simulink library "lib_methods"  (Simulink 7.7)
settings: Solver=ode45  StartTime=0.0  StopTime=10.0  RelTol=1e-3
undefined symbols (not defined in the file): AOBC_dt, DiscIntNeverNeededParam, dt, I, mom_lim, MTQ_out, Ratelim, RW_J, target_mom, three_one_skew_matrix, UT1_UTC
libraries: aerolibutil x15, lib_util x15, vrlib x4, lib_astrodynamics x3, aerolibtransform2 x1, lib_methods x1, lib_env x1
(part 1 of 2)
settings Model: Creator=miyata  LastModifiedBy=yamaurashusaku

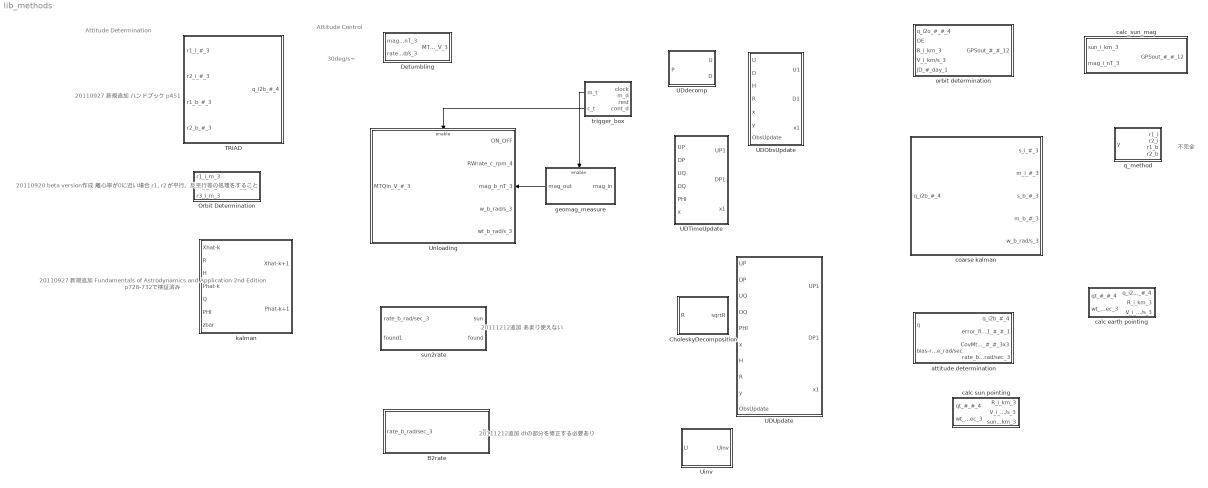
== system lib_methods ==
  note: Attitude Determination
  note: Attitude Control
  note: 30deg/s~
  note: 20110920 beta version作成
      | 離心率が0に近い場合
      | r1, r2が平行、反平行等の処理をすること
  note: 20110927 新規追加
      | ハンドブック p451
  note: 20110927 新規追加
      | Fundamentals of Astrodynamics and Application
      | 2nd Edition p728-732で検証済み
  note: 20111212追加
      | あまり使えない
  note: 20111212追加
      | dtの部分を修正する必要あり
  note: 不完全
  B2rate : Subsystem
  CholeskyDecomposition : Stateflow chart  TreatAsAtomicUnit=on
  Detumbling : Subsystem
  Orbit Determination : Subsystem
  TRIAD : Subsystem
  UDObsUpdate : Stateflow chart  TreatAsAtomicUnit=on
  UDTimeUpdate : Stateflow chart  TreatAsAtomicUnit=on
  UDUpdate : Stateflow chart  TreatAsAtomicUnit=on
  UDdecomp : Stateflow chart  TreatAsAtomicUnit=on
  Uinv : Stateflow chart  TreatAsAtomicUnit=on
  Unloading : Subsystem  TreatAsAtomicUnit=on
  attitude determination : Subsystem
  calc earth pointing : Subsystem
  calc sun pointing : Subsystem
  calc_sun_mag : Subsystem
  coarse kalman : Subsystem
  geomag_measure : Subsystem  TreatAsAtomicUnit=on
  kalman : Subsystem
  orbit determination : Subsystem
  q_method : Stateflow chart  TreatAsAtomicUnit=on
  sun2rate : Subsystem
  trigger_box : Stateflow chart  TreatAsAtomicUnit=on
  wires:
  geomag_measure/1(mag_out) -> Unloading/3(mag_b_nT_3)
  trigger_box/2(c_t) -> Unloading/Enable
  trigger_box/1(m_t) -> geomag_measure/Enable

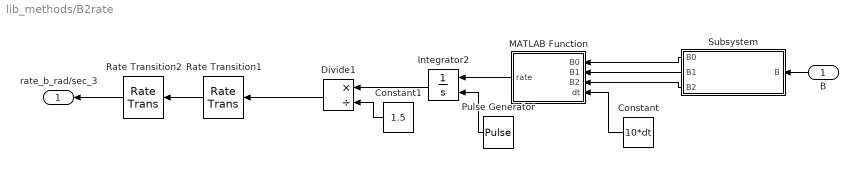
== system lib_methods/B2rate ==
  B : Inport
  Constant : Constant  Value=10*dt
  Constant1 : Constant  Value=1.5
  Divide1 : Product  Inputs=*/
  Integrator2 : Integrator  ExternalReset=rising
  MATLAB Function : Stateflow chart  TreatAsAtomicUnit=on
  Pulse Generator : DiscretePulseGenerator  PulseType=Time based  Period=1.5  PulseWidth=10  PhaseDelay=dt
  Rate Transition1 : RateTransition  Deterministic=off  OutPortSampleTime=1.5
  Rate Transition2 : RateTransition  Deterministic=off  OutPortSampleTime=0
  Subsystem : Subsystem
  rate_b_rad/sec_3 : Outport
  wires:
  MATLAB Function/1(rate) -> Integrator2/1
  Constant/1 -> MATLAB Function/4(dt)
  Subsystem/1(B0) -> MATLAB Function/1(B0)
  Subsystem/2(B1) -> MATLAB Function/2(B1)
  Subsystem/3(B2) -> MATLAB Function/3(B2)
  Pulse Generator/1 -> Integrator2/2
  Divide1/1 -> Rate Transition1/1
  Integrator2/1 -> Divide1/1
  Constant1/1 -> Divide1/2
  Rate Transition1/1 -> Rate Transition2/1
  Rate Transition2/1 -> rate_b_rad/sec_3/1
  B/1 -> Subsystem/1(B)

== system lib_methods/Detumbling ==
  mag_b_nT_3 : Inport
  rate_b_rad/s_3 : Inport  Port=2
  Clock : Clock
      settings: Decimation=10
  Detumbling : Stateflow chart  TreatAsAtomicUnit=on
  Memory : Memory
  MTQvol_b_V_3 : Outport
  wires:
  Detumbling/1(d) -> MTQvol_b_V_3/1
  Memory/1 -> Detumbling/2(mag_b_old)
  Clock/1 -> Detumbling/4(time)
  rate_b_rad/s_3/1 -> Detumbling/3(rate_b)
  mag_b_nT_3/1 -> Detumbling/1(mag_b), Memory/1

== system lib_methods/Orbit Determination ==
  r1_i_m_3 : Inport
  r2_i_m_3 : Inport  Port=2
  r3_i_m_3 : Inport  Port=3
  MATLAB Function : Stateflow chart  TreatAsAtomicUnit=on
  OE_i_#_6 : Outport
  wires:
  MATLAB Function/1(OE) -> OE_i_#_6/1
  r3_i_m_3/1 -> MATLAB Function/3(r3)
  r2_i_m_3/1 -> MATLAB Function/2(r2)
  r1_i_m_3/1 -> MATLAB Function/1(r1)

== system lib_methods/TRIAD ==
  r1_i_#_3 : Inport
  r2_i_#_3 : Inport  Port=2
  r1_b_#_3 : Inport  Port=3
  r2_b_#_3 : Inport  Port=4
  Direction Cosine Matrix  to Quaternions : aerolibtransform2/Direction Cosine Matrix  to Quaternions
  MATLAB Function : Stateflow chart  TreatAsAtomicUnit=on
  Quaternion Normalize : aerolibutil/Quaternion Normalize
  q_i2b_#_4 : Outport
  wires:
  r2_b_#_3/1 -> MATLAB Function/4(w2)
  r1_b_#_3/1 -> MATLAB Function/3(w1)
  r2_i_#_3/1 -> MATLAB Function/2(v2)
  r1_i_#_3/1 -> MATLAB Function/1(v1)
  Direction Cosine Matrix  to Quaternions/1 -> Quaternion Normalize/1
  Quaternion Normalize/1 -> q_i2b_#_4/1
  MATLAB Function/1(A) -> Direction Cosine Matrix  to Quaternions/1

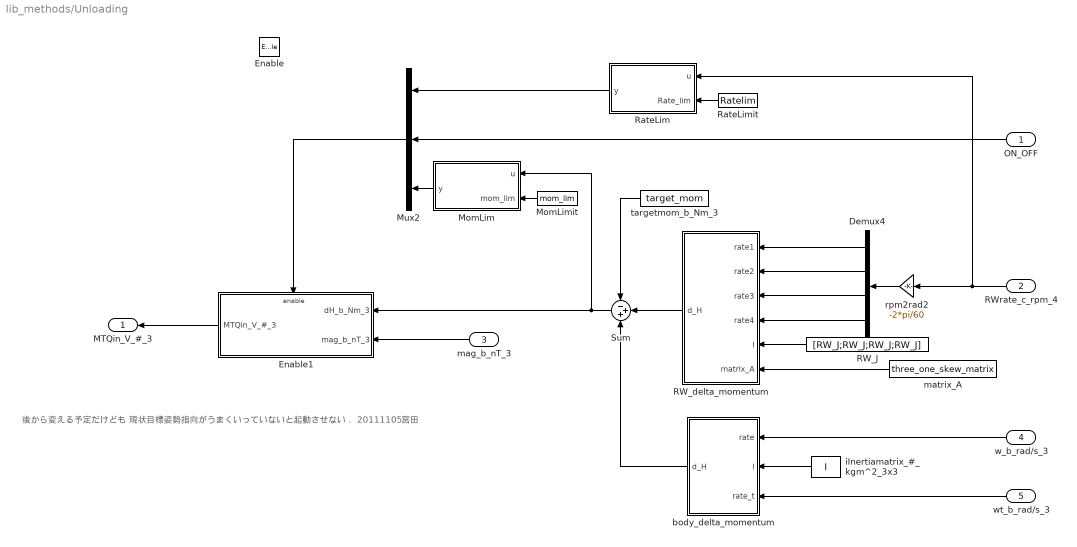
== system lib_methods/Unloading ==
  note: 後から変える予定だけども
      | 現状目標姿勢指向がうまくいっていないと起動させない．
      | 20111105宮田
  ON_OFF : Inport
  RWrate_c_rpm_4 : Inport  Port=2
  mag_b_nT_3 : Inport  Port=3
  w_b_rad/s_3 : Inport  Port=4
  wt_b_rad/s_3 : Inport  Port=5
  Enable : EnablePort  StatesWhenEnabling=reset
  Demux4 : Demux
  Enable1 : Subsystem  TreatAsAtomicUnit=on
  MomLim : Stateflow chart  TreatAsAtomicUnit=on
  MomLimit : Constant  Value=mom_lim
  Mux2 : Mux  Inputs=3
  RW_J : Constant  Value=[RW_J;RW_J;RW_J;RW_J]
  RW_delta_momentum : Stateflow chart  TreatAsAtomicUnit=on
  RateLim : Stateflow chart  TreatAsAtomicUnit=on
  RateLimit : Constant  Value=Ratelim
  Sum : Sum  Inputs=-++
  body_delta_momentum : Stateflow chart  TreatAsAtomicUnit=on
  iInertiamatrix_#_kgm^2_3x3 : Constant  Value=I
  matrix_A : Constant  Value=three_one_skew_matrix
  rpm2rad2 : Gain  Gain=-2*pi/60
  targetmom_b_Nm_3 : Constant  Value=target_mom
  MTQin_V_#_3 : Outport  OutputWhenDisabled=reset  InitialOutput=[0;0;0]
  wires:
  RW_delta_momentum/1(d_H) -> Sum/2
  body_delta_momentum/1(d_H) -> Sum/3
  Demux4/1 -> RW_delta_momentum/1(rate1)
  Demux4/2 -> RW_delta_momentum/2(rate2)
  Demux4/3 -> RW_delta_momentum/3(rate3)
  Demux4/4 -> RW_delta_momentum/4(rate4)
  RWrate_c_rpm_4/1 -> rpm2rad2/1, RateLim/1(u)
  rpm2rad2/1 -> Demux4/1
  wt_b_rad/s_3/1 -> body_delta_momentum/3(rate_t)
  Sum/1 -> MomLim/1(u), Enable1/1(dH_b_Nm_3)
  Enable1/1(MTQin_V_#_3) -> MTQin_V_#_3/1
  w_b_rad/s_3/1 -> body_delta_momentum/1(rate)
  Mux2/1 -> Enable1/Enable
  RateLim/1(y) -> Mux2/1
  RateLimit/1 -> RateLim/2(Rate_lim)
  ON_OFF/1 -> Mux2/2
  MomLim/1(y) -> Mux2/3
  MomLimit/1 -> MomLim/2(mom_lim)
  targetmom_b_Nm_3/1 -> Sum/1
  RW_J/1 -> RW_delta_momentum/5(I)
  iInertiamatrix_#_kgm^2_3x3/1 -> body_delta_momentum/2(I)
  matrix_A/1 -> RW_delta_momentum/6(matrix_A)
  mag_b_nT_3/1 -> Enable1/2(mag_b_nT_3)

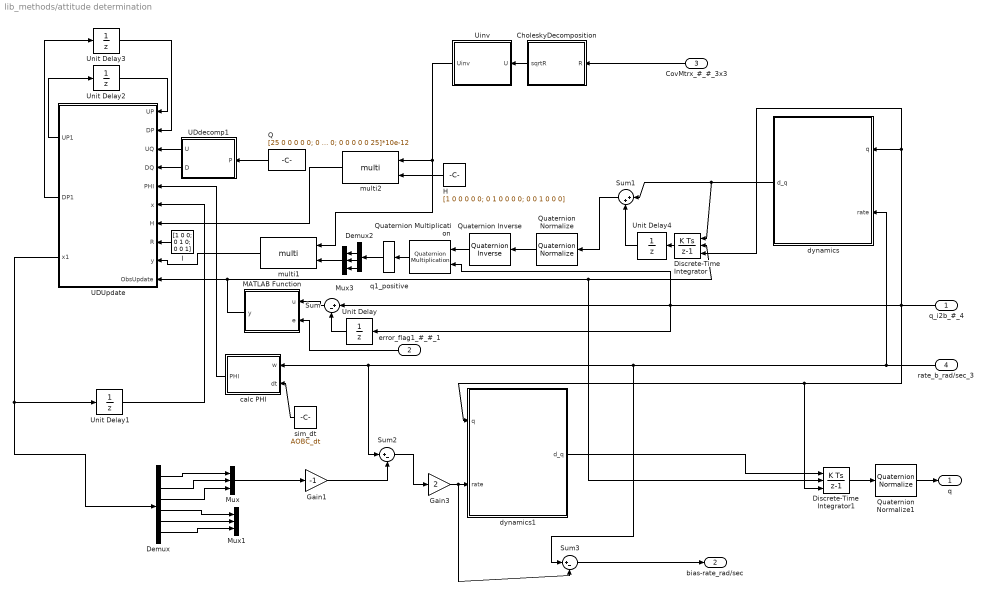
== system lib_methods/attitude determination ==
  q_i2b_#_4 : Inport
  error_flag1_#_#_1 : Inport  Port=2
  CovMtrx_#_#_3x3 : Inport  Port=3
  rate_b_rad/sec_3 : Inport  Port=4
  CholeskyDecomposition : Stateflow chart  TreatAsAtomicUnit=on
  Demux : Demux  Outputs=6
  Demux2 : Demux
  Discrete-Time Integrator : DiscreteIntegrator  ExternalReset=rising  InitialConditionSource=external  SampleTime=-1  ICPrevOutput=DiscIntNeverNeededParam  ICPrevScaledInput=DiscIntNeverNeededParam
  Discrete-Time Integrator1 : DiscreteIntegrator  ExternalReset=rising  InitialConditionSource=external  SampleTime=-1  ICPrevOutput=DiscIntNeverNeededParam  ICPrevScaledInput=DiscIntNeverNeededParam
  Gain1 : Gain  Gain=-1
  Gain3 : Gain  Gain=2
  H : Constant  Value=[1 0 0 0 0 0; 0 1 0 0 0 0; 0 0 1 0 0 0]  VectorParams1D=off
  I : Constant  Value=[1 0 0; 0 1 0; 0 0 1]
  MATLAB Function : Stateflow chart  TreatAsAtomicUnit=on
  Mux : Mux  Inputs=3
  Mux1 : Mux  Inputs=3
  Mux3 : Mux  Inputs=3
  Q : Constant  Value=[25 0 0 0 0 0; 0 25 0 0 0 0; 0 0 25 0 0 0; 0 0 0 25 0 0; 0 0 0 0 25 0; 0 0 0 0 0 25]*10e-12
  Quaternion Inverse : aerolibutil/Quaternion Inverse
  Quaternion Multiplication : aerolibutil/Quaternion Multiplication
  Quaternion Normalize : aerolibutil/Quaternion Normalize
  Quaternion Normalize1 : aerolibutil/Quaternion Normalize
  Sum : Sum  Inputs=|+-
  Sum1 : Sum  Inputs=|++
  Sum2 : Sum  Inputs=|+-
  Sum3 : Sum  Inputs=|+-
  UDUpdate : Stateflow chart  TreatAsAtomicUnit=on
  UDdecomp1 : Stateflow chart  TreatAsAtomicUnit=on
  Uinv : Stateflow chart  TreatAsAtomicUnit=on
  Unit Delay : UnitDelay  X0=[1 0 0 0]  SampleTime=AOBC_dt
  Unit Delay1 : UnitDelay  X0=[1; 2; 3; 4; 5; 6]  SampleTime=AOBC_dt
  Unit Delay2 : UnitDelay  X0=[1 2 3 4 5 6; 0 1 2 3 4 5; 0 0 1 2 3 4; 0 0 0 1 2 3; 0 0 0 0 1 2; 0 0 0 0 0 1]  SampleTime=AOBC_dt
  Unit Delay3 : UnitDelay  X0=[10 0 0 0 0 0; 0 10 0 0 0 0; 0 0 10 0 0 0; 0 0 0 10 0 0; 0 0 0 0 10 0; 0 0 0 0 0 10]  SampleTime=AOBC_dt
  Unit Delay4 : UnitDelay  X0=[1 0 0 0]  SampleTime=AOBC_dt
  calc PHI : Stateflow chart  TreatAsAtomicUnit=on
  dynamics : Stateflow chart  TreatAsAtomicUnit=on
  dynamics1 : Stateflow chart  TreatAsAtomicUnit=on
  multi1 : lib_util/multi
  multi2 : lib_util/multi
  q1_positive : lib_util/q1_positive
  sim_dt : Constant  Value=AOBC_dt
  q : Outport
  bias-rate_rad/sec : Outport  Port=2
  wires:
  UDUpdate/3(x1) -> Unit Delay1/1, Demux/1
  Unit Delay1/1 -> UDUpdate/6(x)
  sim_dt/1 -> calc PHI/2(dt)
  calc PHI/1(PHI) -> UDUpdate/5(PHI)
  UDdecomp1/2(D) -> UDUpdate/4(DQ)
  UDdecomp1/1(U) -> UDUpdate/3(UQ)
  Q/1 -> UDdecomp1/1(P)
  UDUpdate/2(DP1) -> Unit Delay3/1
  UDUpdate/1(UP1) -> Unit Delay2/1
  Unit Delay2/1 -> UDUpdate/1(UP)
  Unit Delay3/1 -> UDUpdate/2(DP)
  MATLAB Function/1(y) -> UDUpdate/10(ObsUpdate), Discrete-Time Integrator/2, Discrete-Time Integrator1/2
  Sum/1 -> MATLAB Function/1(u)
  Unit Delay/1 -> Sum/2
  q_i2b_#_4/1 -> dynamics1/1(q), Discrete-Time Integrator1/3, dynamics/1(q), Discrete-Time Integrator/3, Unit Delay/1, Quaternion Multiplication/2, Sum/1
  Demux2/2 -> Mux3/1
  Demux2/3 -> Mux3/2
  Demux2/4 -> Mux3/3
  q1_positive/1 -> Demux2/1
  dynamics/1(d_q) -> Discrete-Time Integrator/1, Sum1/1
  Discrete-Time Integrator/1 -> Unit Delay4/1
  Quaternion Normalize/1 -> Quaternion Inverse/1
  Quaternion Multiplication/1 -> q1_positive/1
  Quaternion Inverse/1 -> Quaternion Multiplication/1
  Unit Delay4/1 -> Sum1/2
  Sum1/1 -> Quaternion Normalize/1
  rate_b_rad/sec_3/1 -> dynamics/2(rate), calc PHI/1(w), Sum2/1, Sum3/1
  Gain1/1 -> Sum2/2
  Discrete-Time Integrator1/1 -> Quaternion Normalize1/1
  Quaternion Normalize1/1 -> q/1
  Sum2/1 -> Gain3/1
  dynamics1/1(d_q) -> Discrete-Time Integrator1/1
  Gain3/1 -> dynamics1/2(rate), Sum3/2
  CovMtrx_#_#_3x3/1 -> CholeskyDecomposition/1(R)
  Demux/1 -> Mux/1
  Demux/2 -> Mux/2
  Demux/3 -> Mux/3
  Demux/4 -> Mux1/1
  Demux/5 -> Mux1/2
  Demux/6 -> Mux1/3
  Mux/1 -> Gain1/1
  CholeskyDecomposition/1(sqrtR) -> Uinv/1(U)
  I/1 -> UDUpdate/8(R)
  Uinv/1(Uinv) -> multi2/1, multi1/1
  H/1 -> multi2/2
  multi2/1 -> UDUpdate/7(H)
  Mux3/1 -> multi1/2
  multi1/1 -> UDUpdate/9(y)
  Sum3/1 -> bias-rate_rad/sec/1
  error_flag1_#_#_1/1 -> MATLAB Function/2(e)

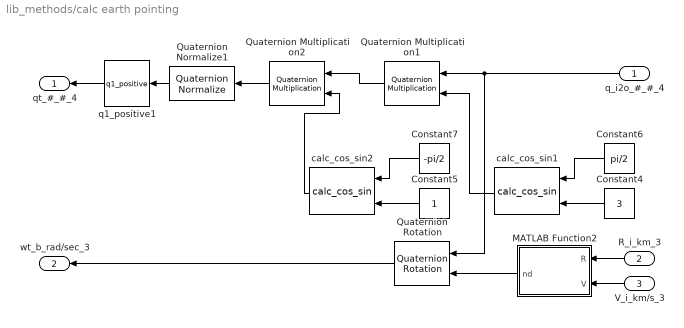
== system lib_methods/calc earth pointing ==
  q_i2o_#_#_4 : Inport
  R_i_km_3 : Inport  Port=2
  V_i_km/s_3 : Inport  Port=3
  Constant4 : Constant  Value=3
  Constant5 : Constant
  Constant6 : Constant  Value=pi/2
  Constant7 : Constant  Value=-pi/2
  MATLAB Function2 : Stateflow chart  TreatAsAtomicUnit=on
  Quaternion Multiplication1 : aerolibutil/Quaternion Multiplication
  Quaternion Multiplication2 : aerolibutil/Quaternion Multiplication
  Quaternion Normalize1 : aerolibutil/Quaternion Normalize
  Quaternion Rotation : aerolibutil/Quaternion Rotation
  calc_cos_sin1 : lib_util/calc_cos_sin
  calc_cos_sin2 : lib_util/calc_cos_sin
  q1_positive1 : lib_util/q1_positive
  qt_#_#_4 : Outport
  wt_b_rad/sec_3 : Outport  Port=2
  wires:
  Constant4/1 -> calc_cos_sin1/2
  Constant6/1 -> calc_cos_sin1/1
  Constant5/1 -> calc_cos_sin2/2
  Constant7/1 -> calc_cos_sin2/1
  q_i2o_#_#_4/1 -> Quaternion Multiplication1/1, Quaternion Rotation/1
  calc_cos_sin1/1 -> Quaternion Multiplication1/2
  Quaternion Multiplication1/1 -> Quaternion Multiplication2/1
  calc_cos_sin2/1 -> Quaternion Multiplication2/2
  Quaternion Multiplication2/1 -> Quaternion Normalize1/1
  Quaternion Normalize1/1 -> q1_positive1/1
  q1_positive1/1 -> qt_#_#_4/1
  MATLAB Function2/1(nd) -> Quaternion Rotation/2
  Quaternion Rotation/1 -> wt_b_rad/sec_3/1
  R_i_km_3/1 -> MATLAB Function2/1(R)
  V_i_km/s_3/1 -> MATLAB Function2/2(V)

== system lib_methods/calc sun pointing ==
  R_i_km_3 : Inport
  V_i_km/s_3 : Inport  Port=2
  sun_i_km_3 : Inport  Port=3
  Constant : Constant  Value=[0; 0; 0]
  MATLAB Function1 : Stateflow chart  TreatAsAtomicUnit=on
  TRIAD : lib_methods/TRIAD
  qt_#_#_4 : Outport
  wt_b_rad/sec_3 : Outport  Port=2
  wires:
  R_i_km_3/1 -> MATLAB Function1/1(R)
  V_i_km/s_3/1 -> MATLAB Function1/2(V)
  sun_i_km_3/1 -> MATLAB Function1/3(S)
  MATLAB Function1/1(n1) -> TRIAD/1
  MATLAB Function1/2(n2) -> TRIAD/2
  MATLAB Function1/3(y) -> TRIAD/3
  MATLAB Function1/4(z) -> TRIAD/4
  TRIAD/1 -> qt_#_#_4/1
  Constant/1 -> wt_b_rad/sec_3/1

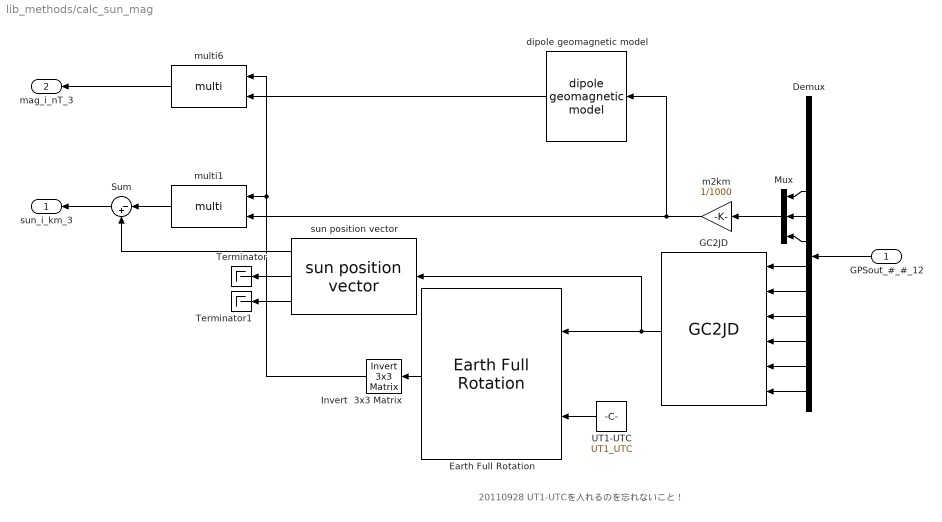
== system lib_methods/calc_sun_mag ==
  note: 20110928 UT1-UTCを入れるのを忘れないこと！
  GPSout_#_#_12 : Inport
  Demux : Demux  Outputs=12
  Earth Full Rotation : lib_astrodynamics/Earth Full Rotation
  GC2JD : lib_util/GC2JD
  Invert  3x3 Matrix : aerolibutil/Invert  3x3 Matrix
  Mux : Mux  Inputs=3
  Sum : Sum  Inputs=|-+
  Terminator : Terminator
  Terminator1 : Terminator
  UT1-UTC : Constant  Value=UT1_UTC
  dipole geomagnetic model : lib_env/dipole geomagnetic model
  m2km : Gain  Gain=1/1000
  multi1 : lib_util/multi
  multi6 : lib_util/multi
  sun position vector : lib_astrodynamics/sun position vector
  sun_i_km_3 : Outport
  mag_i_nT_3 : Outport  Port=2
  wires:
  Sum/1 -> sun_i_km_3/1
  multi1/1 -> Sum/1
  sun position vector/1 -> Sum/2
  multi6/1 -> mag_i_nT_3/1
  sun position vector/3 -> Terminator1/1
  sun position vector/2 -> Terminator/1
  m2km/1 -> multi1/2, dipole geomagnetic model/1
  Invert  3x3 Matrix/1 -> multi1/1, multi6/1
  Earth Full Rotation/1 -> Invert  3x3 Matrix/1
  Mux/1 -> m2km/1
  Demux/6 -> Mux/3
  Demux/5 -> Mux/2
  Demux/4 -> Mux/1
  UT1-UTC/1 -> Earth Full Rotation/2
  GC2JD/1 -> sun position vector/1, Earth Full Rotation/1
  Demux/7 -> GC2JD/1
  Demux/8 -> GC2JD/2
  Demux/9 -> GC2JD/3
  Demux/10 -> GC2JD/4
  Demux/11 -> GC2JD/5
  Demux/12 -> GC2JD/6
  GPSout_#_#_12/1 -> Demux/1
  dipole geomagnetic model/1 -> multi6/2

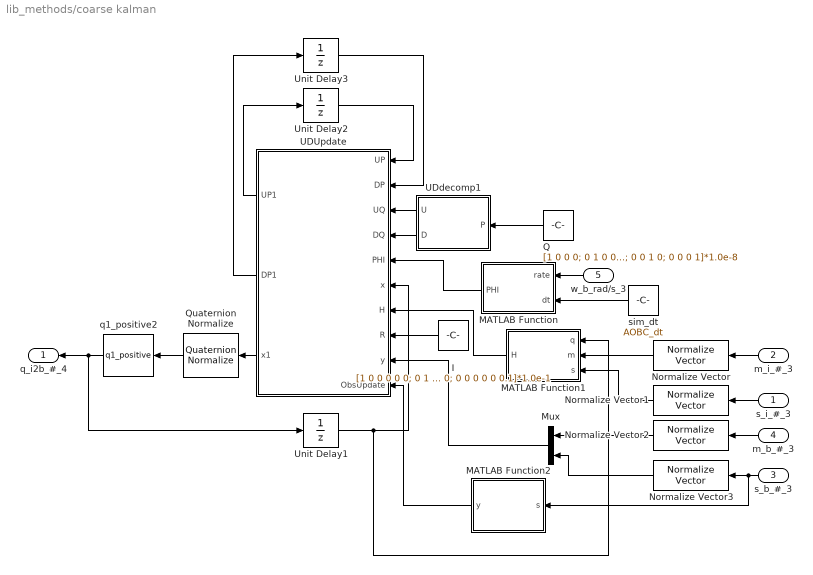
== system lib_methods/coarse kalman ==
  s_i_#_3 : Inport
  m_i_#_3 : Inport  Port=2
  s_b_#_3 : Inport  Port=3
  m_b_#_3 : Inport  Port=4
  w_b_rad/s_3 : Inport  Port=5
  I : Constant  Value=[1 0 0 0 0 0; 0 1 0 0 0 0; 0 0 1 0 0 0; 0 0 0 0.1 0 0; 0 0 0 0 0.1 0; 0 0 0 0 0 0.1]*1.0e-1
  MATLAB Function : Stateflow chart  TreatAsAtomicUnit=on
  MATLAB Function1 : Stateflow chart  TreatAsAtomicUnit=on
  MATLAB Function2 : Stateflow chart  TreatAsAtomicUnit=on
  Mux : Mux  Inputs=2
  Normalize Vector{,1..3} (4 alike) : vrlib/Utilities/Normalize Vector  maxzero=0
  Q : Constant  Value=[1 0 0 0; 0 1 0 0; 0 0 1 0; 0 0 0 1]*1.0e-8
  Quaternion Normalize : aerolibutil/Quaternion Normalize
  UDUpdate : Stateflow chart  TreatAsAtomicUnit=on
  UDdecomp1 : Stateflow chart  TreatAsAtomicUnit=on
  Unit Delay1 : UnitDelay  X0=[1; 0; 0; 0]  SampleTime=AOBC_dt
  Unit Delay2 : UnitDelay  X0=[1 0 0 0; 0 1 0 0; 0 0 1 0; 0 0 0 1]  SampleTime=AOBC_dt
  Unit Delay3 : UnitDelay  X0=[0.5 0 0 0; 0 0.5 0 0; 0 0 0.5 0; 0 0 0 0.5]  SampleTime=AOBC_dt
  q1_positive2 : lib_util/q1_positive
  sim_dt : Constant  Value=AOBC_dt
  q_i2b_#_4 : Outport
  wires:
  UDUpdate/1(UP1) -> Unit Delay2/1
  Unit Delay2/1 -> UDUpdate/1(UP)
  Unit Delay3/1 -> UDUpdate/2(DP)
  UDUpdate/2(DP1) -> Unit Delay3/1
  Q/1 -> UDdecomp1/1(P)
  UDdecomp1/1(U) -> UDUpdate/3(UQ)
  UDdecomp1/2(D) -> UDUpdate/4(DQ)
  I/1 -> UDUpdate/8(R)
  Unit Delay1/1 -> UDUpdate/6(x), MATLAB Function1/1(q)
  UDUpdate/3(x1) -> Quaternion Normalize/1
  w_b_rad/s_3/1 -> MATLAB Function/1(rate)
  sim_dt/1 -> MATLAB Function/2(dt)
  MATLAB Function/1(PHI) -> UDUpdate/5(PHI)
  MATLAB Function1/1(H) -> UDUpdate/7(H)
  m_i_#_3/1 -> Normalize Vector/1
  s_i_#_3/1 -> Normalize Vector1/1
  m_b_#_3/1 -> Normalize Vector2/1
  s_b_#_3/1 -> Normalize Vector3/1, MATLAB Function2/1(s)
  MATLAB Function2/1(y) -> UDUpdate/10(ObsUpdate)
  Normalize Vector/1 -> MATLAB Function1/2(m)
  Normalize Vector1/1 -> MATLAB Function1/3(s)
  q1_positive2/1 -> q_i2b_#_4/1, Unit Delay1/1
  Normalize Vector2/1 -> Mux/1
  Normalize Vector3/1 -> Mux/2
  Mux/1 -> UDUpdate/9(y)
  Quaternion Normalize/1 -> q1_positive2/1

== system lib_methods/geomag_measure ==
  mag_in : Inport
  Enable : EnablePort  StatesWhenEnabling=reset
  mag_out : Outport  InitialOutput=[0;0;0]
  wires:
  mag_in/1 -> mag_out/1

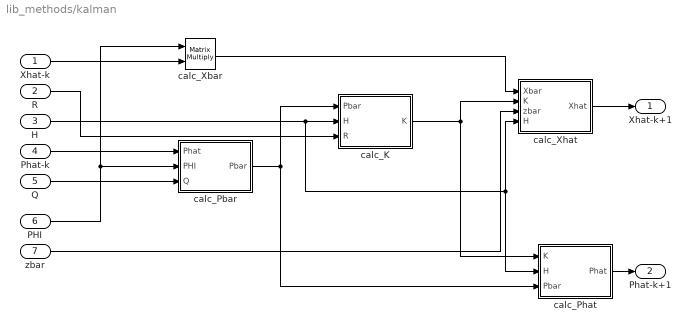
== system lib_methods/kalman ==
  Xhat-k : Inport
  R : Inport  Port=2
  H : Inport  Port=3
  Phat-k : Inport  Port=4
  Q : Inport  Port=5
  PHI : Inport  Port=6
  zbar : Inport  Port=7
  calc_K : Stateflow chart  TreatAsAtomicUnit=on
  calc_Pbar : Stateflow chart  TreatAsAtomicUnit=on
  calc_Phat : Stateflow chart  TreatAsAtomicUnit=on
  calc_Xbar : Product  Multiplication=Matrix(*)  RndMeth=Zero
  calc_Xhat : Stateflow chart  TreatAsAtomicUnit=on
  Xhat-k+1 : Outport
  Phat-k+1 : Outport  Port=2
  wires:
  PHI/1 -> calc_Pbar/2(PHI), calc_Xbar/1
  calc_Xbar/1 -> calc_Xhat/1(Xbar)
  calc_Pbar/1(Pbar) -> calc_K/1(Pbar), calc_Phat/3(Pbar)
  H/1 -> calc_Phat/2(H), calc_Xhat/4(H), calc_K/2(H)
  calc_K/1(K) -> calc_Xhat/2(K), calc_Phat/1(K)
  Xhat-k/1 -> calc_Xbar/2
  calc_Xhat/1(Xhat) -> Xhat-k+1/1
  R/1 -> calc_K/3(R)
  Phat-k/1 -> calc_Pbar/1(Phat)
  Q/1 -> calc_Pbar/3(Q)
  calc_Phat/1(Phat) -> Phat-k+1/1
  zbar/1 -> calc_Xhat/3(zbar)

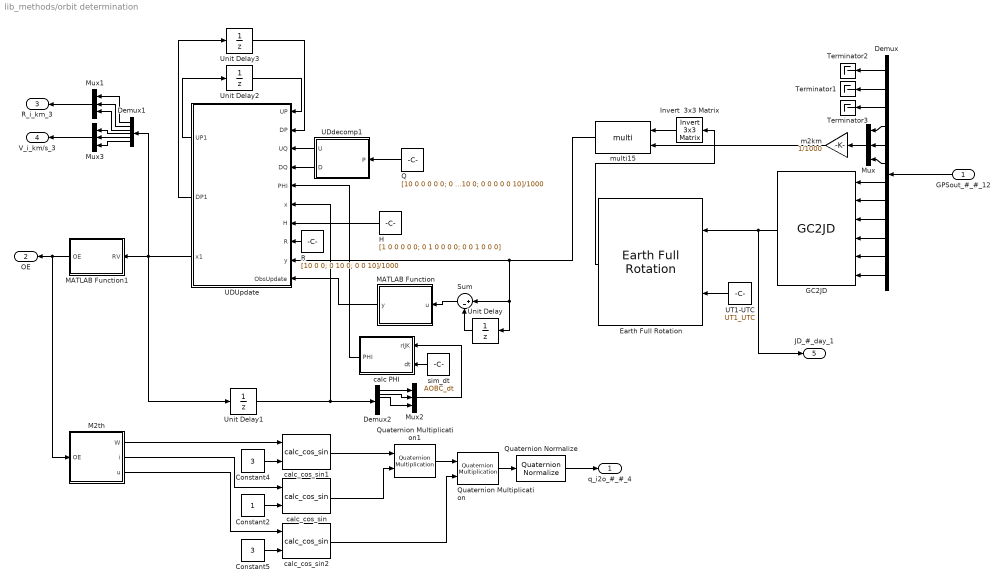
== system lib_methods/orbit determination ==
  GPSout_#_#_12 : Inport
  Constant2 : Constant
  Constant4 : Constant  Value=3
  Constant5 : Constant  Value=3
  Demux : Demux  Outputs=12
  Demux1 : Demux  Outputs=6
  Demux2 : Demux  Outputs=6
  Earth Full Rotation : lib_astrodynamics/Earth Full Rotation
  GC2JD : lib_util/GC2JD
  H : Constant  Value=[1 0 0 0 0 0; 0 1 0 0 0 0; 0 0 1 0 0 0]  VectorParams1D=off
  Invert  3x3 Matrix : aerolibutil/Invert  3x3 Matrix
  M2th : Stateflow chart  TreatAsAtomicUnit=on
  MATLAB Function : Stateflow chart  TreatAsAtomicUnit=on
  MATLAB Function1 : Stateflow chart  TreatAsAtomicUnit=on
  Mux{,1..3} (4 alike) : Mux  Inputs=3
  Q : Constant  Value=[10 0 0 0 0 0; 0 10 0 0 0 0; 0 0 10 0 0 0; 0 0 0 10 0 0; 0 0 0 0 10 0; 0 0 0 0 0 10]/1000
  Quaternion Multiplication : aerolibutil/Quaternion Multiplication
  Quaternion Multiplication1 : aerolibutil/Quaternion Multiplication
  Quaternion Normalize : aerolibutil/Quaternion Normalize
  R : Constant  Value=[10 0 0; 0 10 0; 0 0 10]/1000
  Sum : Sum  Inputs=|+-
  Terminator1 : Terminator
  Terminator2 : Terminator
  Terminator3 : Terminator
  UDUpdate : Stateflow chart  TreatAsAtomicUnit=on
  UDdecomp1 : Stateflow chart  TreatAsAtomicUnit=on
  UT1-UTC : Constant  Value=UT1_UTC
  Unit Delay : UnitDelay  X0=[7000; 0; 0]  SampleTime=AOBC_dt
  Unit Delay1 : UnitDelay  X0=[7000; 7000; 7000; 7; 7; 7]  SampleTime=AOBC_dt
  Unit Delay2 : UnitDelay  X0=[1 2 3 4 5 6; 0 1 2 3 4 5; 0 0 1 2 3 4; 0 0 0 1 2 3; 0 0 0 0 1 2; 0 0 0 0 0 1]  SampleTime=AOBC_dt
  Unit Delay3 : UnitDelay  X0=[10 0 0 0 0 0; 0 10 0 0 0 0; 0 0 10 0 0 0; 0 0 0 10 0 0; 0 0 0 0 10 0; 0 0 0 0 0 10]  SampleTime=AOBC_dt
  calc PHI : Stateflow chart  TreatAsAtomicUnit=on
  calc_cos_sin : lib_util/calc_cos_sin
  calc_cos_sin1 : lib_util/calc_cos_sin
  calc_cos_sin2 : lib_util/calc_cos_sin
  m2km : Gain  Gain=1/1000
  multi15 : lib_util/multi
  sim_dt : Constant  Value=AOBC_dt
  q_i2o_#_#_4 : Outport
  OE : Outport  Port=2
  R_i_km_3 : Outport  Port=3
  V_i_km/s_3 : Outport  Port=4
  JD_#_day_1 : Outport  Port=5
  wires:
  GPSout_#_#_12/1 -> Demux/1
  Demux/12 -> GC2JD/6
  Demux/11 -> GC2JD/5
  Demux/10 -> GC2JD/4
  Demux/9 -> GC2JD/3
  Demux/8 -> GC2JD/2
  Demux/7 -> GC2JD/1
  GC2JD/1 -> Earth Full Rotation/1, JD_#_day_1/1
  UT1-UTC/1 -> Earth Full Rotation/2
  Demux/4 -> Mux/1
  Demux/5 -> Mux/2
  Demux/6 -> Mux/3
  Demux/1 -> Terminator2/1
  Demux/2 -> Terminator1/1
  Demux/3 -> Terminator3/1
  Mux/1 -> m2km/1
  m2km/1 -> multi15/2
  multi15/1 -> Sum/1, Unit Delay/1, UDUpdate/9(y)
  Earth Full Rotation/1 -> Invert  3x3 Matrix/1
  Invert  3x3 Matrix/1 -> multi15/1
  Unit Delay/1 -> Sum/2
  Sum/1 -> MATLAB Function/1(u)
  H/1 -> UDUpdate/7(H)
  Unit Delay3/1 -> UDUpdate/2(DP)
  Unit Delay2/1 -> UDUpdate/1(UP)
  UDUpdate/1(UP1) -> Unit Delay2/1
  UDUpdate/2(DP1) -> Unit Delay3/1
  Q/1 -> UDdecomp1/1(P)
  UDdecomp1/1(U) -> UDUpdate/3(UQ)
  UDdecomp1/2(D) -> UDUpdate/4(DQ)
  calc PHI/1(PHI) -> UDUpdate/5(PHI)
  sim_dt/1 -> calc PHI/2(dt)
  Unit Delay1/1 -> Demux2/1, UDUpdate/6(x)
  Demux2/1 -> Mux2/1
  Demux2/2 -> Mux2/2
  Demux2/3 -> Mux2/3
  Mux2/1 -> calc PHI/1(rIJK)
  UDUpdate/3(x1) -> MATLAB Function1/1(RV), Demux1/1, Unit Delay1/1
  R/1 -> UDUpdate/8(R)
  MATLAB Function1/1(OE) -> M2th/1(OE), OE/1
  calc_cos_sin2/1 -> Quaternion Multiplication/2
  Quaternion Multiplication1/1 -> Quaternion Multiplication/1
  calc_cos_sin/1 -> Quaternion Multiplication1/2
  calc_cos_sin1/1 -> Quaternion Multiplication1/1
  Constant5/1 -> calc_cos_sin2/2
  Constant4/1 -> calc_cos_sin1/2
  Constant2/1 -> calc_cos_sin/2
  Quaternion Multiplication/1 -> Quaternion Normalize/1
  Quaternion Normalize/1 -> q_i2o_#_#_4/1
  Demux1/1 -> Mux1/1
  Demux1/2 -> Mux1/2
  Demux1/3 -> Mux1/3
  Demux1/4 -> Mux3/1
  Demux1/5 -> Mux3/2
  Demux1/6 -> Mux3/3
  Mux3/1 -> V_i_km/s_3/1
  Mux1/1 -> R_i_km_3/1
  M2th/1(W) -> calc_cos_sin1/1
  M2th/2(i) -> calc_cos_sin/1
  M2th/3(u) -> calc_cos_sin2/1
  MATLAB Function/1(y) -> UDUpdate/10(ObsUpdate)

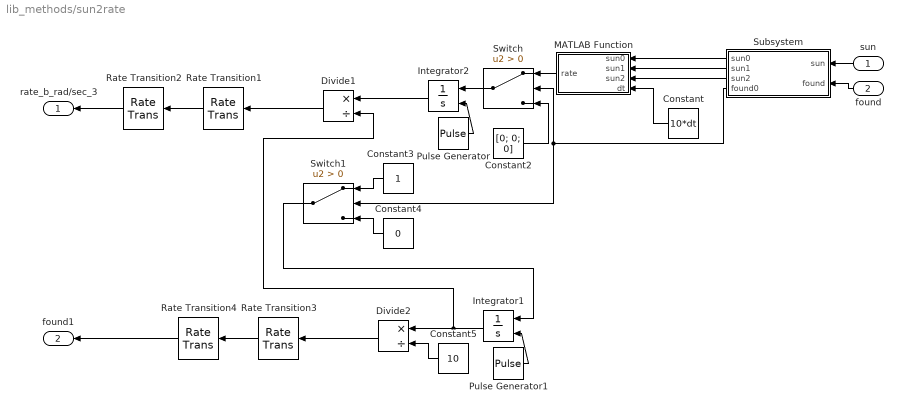
== system lib_methods/sun2rate ==
  sun : Inport
  found : Inport  Port=2
  Constant : Constant  Value=10*dt
  Constant2 : Constant  Value=[0; 0; 0]
  Constant3 : Constant
  Constant4 : Constant  Value=0
  Constant5 : Constant  Value=10
  Divide1 : Product  Inputs=*/
  Divide2 : Product  Inputs=*/
  Integrator1 : Integrator  ExternalReset=rising
  Integrator2 : Integrator  ExternalReset=rising
  MATLAB Function : Stateflow chart  TreatAsAtomicUnit=on
  Pulse Generator : DiscretePulseGenerator  PulseType=Time based  Period=10  PulseWidth=5  PhaseDelay=dt
  Pulse Generator1 : DiscretePulseGenerator  PulseType=Time based  Period=10  PulseWidth=5  PhaseDelay=dt
  Rate Transition1 : RateTransition  Deterministic=off  OutPortSampleTime=10
  Rate Transition2 : RateTransition  Deterministic=off  OutPortSampleTime=0
  Rate Transition3 : RateTransition  Deterministic=off  OutPortSampleTime=10
  Rate Transition4 : RateTransition  Deterministic=off  OutPortSampleTime=0
  Subsystem : Subsystem
  Switch : Switch  Criteria=u2 > Threshold
  Switch1 : Switch  Criteria=u2 > Threshold
  rate_b_rad/sec_3 : Outport
  found1 : Outport  Port=2
  wires:
  Switch1/1 -> Integrator1/1
  Rate Transition4/1 -> found1/1
  Rate Transition3/1 -> Rate Transition4/1
  Constant5/1 -> Divide2/2
  Integrator1/1 -> Divide1/2, Divide2/1
  Divide2/1 -> Rate Transition3/1
  Pulse Generator1/1 -> Integrator1/2
  Constant4/1 -> Switch1/3
  Constant3/1 -> Switch1/1
  Constant2/1 -> Switch/3
  Subsystem/4(found0) -> Switch1/2, Switch/2
  MATLAB Function/1(rate) -> Switch/1
  Switch/1 -> Integrator2/1
  found/1 -> Subsystem/2(found)
  sun/1 -> Subsystem/1(sun)
  Rate Transition2/1 -> rate_b_rad/sec_3/1
  Rate Transition1/1 -> Rate Transition2/1
  Integrator2/1 -> Divide1/1
  Divide1/1 -> Rate Transition1/1
  Pulse Generator/1 -> Integrator2/2
  Subsystem/3(sun2) -> MATLAB Function/3(sun2)
  Subsystem/2(sun1) -> MATLAB Function/2(sun1)
  Subsystem/1(sun0) -> MATLAB Function/1(sun0)
  Constant/1 -> MATLAB Function/4(dt)

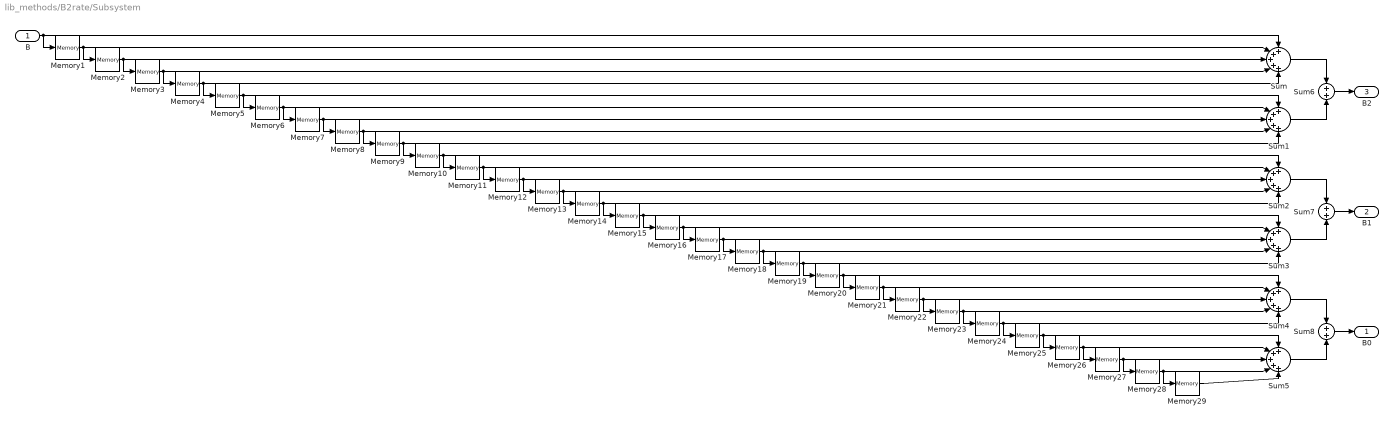
== system lib_methods/B2rate/Subsystem ==
  B : Inport
  Memory{1..29} (29 alike) : Memory  X0=[0;0;0]
  Sum{,1..5} (6 alike) : Sum  Inputs=+++++
  Sum6 : Sum
  Sum7 : Sum
  Sum8 : Sum
  B0 : Outport
  B1 : Outport  Port=2
  B2 : Outport  Port=3
  wires:
  B/1 -> Memory1/1, Sum/1
  Memory1/1 -> Memory2/1, Sum/2
  Memory2/1 -> Memory3/1, Sum/3
  Memory3/1 -> Memory4/1, Sum/4
  Memory4/1 -> Memory5/1, Sum/5
  Memory5/1 -> Memory6/1, Sum1/1
  Memory6/1 -> Memory7/1, Sum1/2
  Memory7/1 -> Memory8/1, Sum1/3
  Memory8/1 -> Memory9/1, Sum1/4
  Memory9/1 -> Memory10/1, Sum1/5
  Memory10/1 -> Memory11/1, Sum2/1
  Memory11/1 -> Memory12/1, Sum2/2
  Memory12/1 -> Memory13/1, Sum2/3
  Memory13/1 -> Memory14/1, Sum2/4
  Memory14/1 -> Memory15/1, Sum2/5
  Memory15/1 -> Memory16/1, Sum3/1
  Memory16/1 -> Memory17/1, Sum3/2
  Memory17/1 -> Memory18/1, Sum3/3
  Memory18/1 -> Memory19/1, Sum3/4
  Memory19/1 -> Memory20/1, Sum3/5
  Memory20/1 -> Memory21/1, Sum4/1
  Memory21/1 -> Memory22/1, Sum4/2
  Memory22/1 -> Memory23/1, Sum4/3
  Memory23/1 -> Memory24/1, Sum4/4
  Memory24/1 -> Memory25/1, Sum4/5
  Memory25/1 -> Memory26/1, Sum5/1
  Memory26/1 -> Memory27/1, Sum5/2
  Memory27/1 -> Memory28/1, Sum5/3
  Memory28/1 -> Memory29/1, Sum5/4
  Memory29/1 -> Sum5/5
  Sum1/1 -> Sum6/2
  Sum/1 -> Sum6/1
  Sum6/1 -> B2/1
  Sum3/1 -> Sum7/2
  Sum2/1 -> Sum7/1
  Sum7/1 -> B1/1
  Sum5/1 -> Sum8/2
  Sum4/1 -> Sum8/1
  Sum8/1 -> B0/1

== system lib_methods/Unloading/Enable1 ==
  dH_b_Nm_3 : Inport
  mag_b_nT_3 : Inport  Port=2
  Enable : EnablePort
  MATLAB Function4 : Stateflow chart  TreatAsAtomicUnit=on
  MTQ_out : Constant  Value=MTQ_out
  MTQin_V_#_3 : Outport  OutputWhenDisabled=reset  InitialOutput=[0;0;0]
  wires:
  MATLAB Function4/1(m) -> MTQin_V_#_3/1
  mag_b_nT_3/1 -> MATLAB Function4/2(mag)
  MTQ_out/1 -> MATLAB Function4/3(max_mag)
  dH_b_Nm_3/1 -> MATLAB Function4/1(dH)

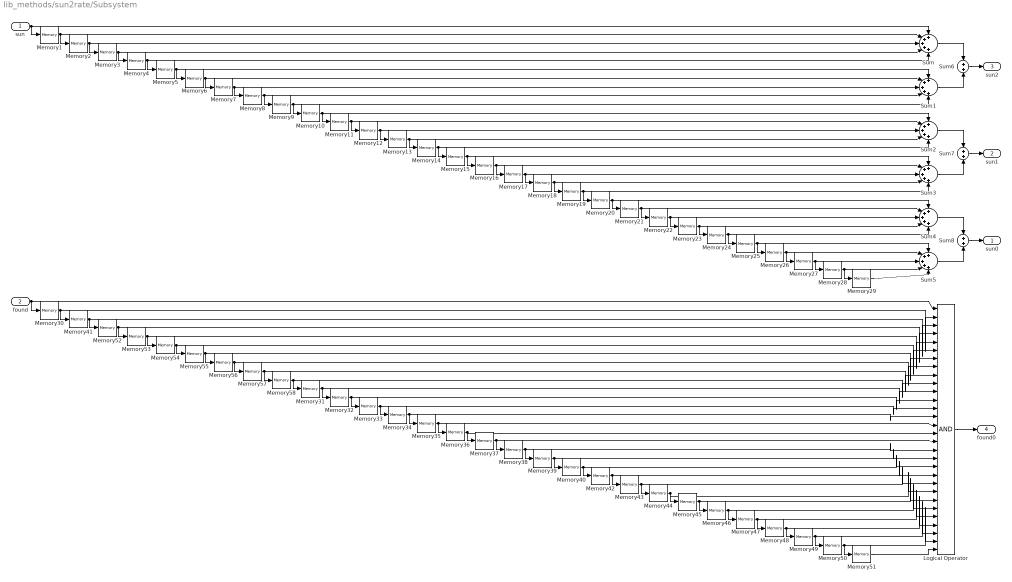
== system lib_methods/sun2rate/Subsystem ==
  sun : Inport
  found : Inport  Port=2
  Logical Operator : Logic  Inputs=30  AllPortsSameDT=off  OutDataTypeStr=boolean
  Memory{1..29} (29 alike) : Memory  X0=[0;0;0]
  Memory{30..58} (29 alike) : Memory
  Sum{,1..5} (6 alike) : Sum  Inputs=+++++
  Sum6 : Sum
  Sum7 : Sum
  Sum8 : Sum
  sun0 : Outport
  sun1 : Outport  Port=2
  sun2 : Outport  Port=3
  found0 : Outport  Port=4
  wires:
  Logical Operator/1 -> found0/1
  Memory51/1 -> Logical Operator/30
  Memory50/1 -> Logical Operator/29, Memory51/1
  Memory49/1 -> Logical Operator/28, Memory50/1
  Memory48/1 -> Logical Operator/27, Memory49/1
  Memory47/1 -> Logical Operator/26, Memory48/1
  Memory46/1 -> Logical Operator/25, Memory47/1
  Memory45/1 -> Logical Operator/24, Memory46/1
  Memory44/1 -> Logical Operator/23, Memory45/1
  Memory43/1 -> Logical Operator/22, Memory44/1
  Memory42/1 -> Logical Operator/21, Memory43/1
  Memory40/1 -> Logical Operator/20, Memory42/1
  Memory39/1 -> Logical Operator/19, Memory40/1
  Memory38/1 -> Logical Operator/18, Memory39/1
  Memory37/1 -> Logical Operator/17, Memory38/1
  Memory36/1 -> Logical Operator/16, Memory37/1
  Memory35/1 -> Logical Operator/15, Memory36/1
  Memory34/1 -> Logical Operator/14, Memory35/1
  Memory33/1 -> Logical Operator/13, Memory34/1
  Memory32/1 -> Logical Operator/12, Memory33/1
  Memory31/1 -> Logical Operator/11, Memory32/1
  Memory58/1 -> Logical Operator/10, Memory31/1
  Memory57/1 -> Logical Operator/9, Memory58/1
  Memory56/1 -> Logical Operator/8, Memory57/1
  Memory55/1 -> Logical Operator/7, Memory56/1
  Memory54/1 -> Logical Operator/6, Memory55/1
  Memory53/1 -> Logical Operator/5, Memory54/1
  Memory52/1 -> Logical Operator/4, Memory53/1
  Memory41/1 -> Logical Operator/3, Memory52/1
  Memory30/1 -> Logical Operator/2, Memory41/1
  found/1 -> Logical Operator/1, Memory30/1
  Sum8/1 -> sun0/1
  Sum4/1 -> Sum8/1
  Sum5/1 -> Sum8/2
  Sum7/1 -> sun1/1
  Sum2/1 -> Sum7/1
  Sum3/1 -> Sum7/2
  Sum6/1 -> sun2/1
  Sum/1 -> Sum6/1
  Sum1/1 -> Sum6/2
  Memory29/1 -> Sum5/5
  Memory28/1 -> Sum5/4, Memory29/1
  Memory27/1 -> Sum5/3, Memory28/1
  Memory26/1 -> Sum5/2, Memory27/1
  Memory25/1 -> Sum5/1, Memory26/1
  Memory24/1 -> Sum4/5, Memory25/1
  Memory23/1 -> Sum4/4, Memory24/1
  Memory22/1 -> Sum4/3, Memory23/1
  Memory21/1 -> Sum4/2, Memory22/1
  Memory20/1 -> Sum4/1, Memory21/1
  Memory19/1 -> Sum3/5, Memory20/1
  Memory18/1 -> Sum3/4, Memory19/1
  Memory17/1 -> Sum3/3, Memory18/1
  Memory16/1 -> Sum3/2, Memory17/1
  Memory15/1 -> Sum3/1, Memory16/1
  Memory14/1 -> Sum2/5, Memory15/1
  Memory13/1 -> Sum2/4, Memory14/1
  Memory12/1 -> Sum2/3, Memory13/1
  Memory11/1 -> Sum2/2, Memory12/1
  Memory10/1 -> Sum2/1, Memory11/1
  Memory9/1 -> Sum1/5, Memory10/1
  Memory8/1 -> Sum1/4, Memory9/1
  Memory7/1 -> Sum1/3, Memory8/1
  Memory6/1 -> Sum1/2, Memory7/1
  Memory5/1 -> Sum1/1, Memory6/1
  Memory4/1 -> Sum/5, Memory5/1
  Memory3/1 -> Sum/4, Memory4/1
  Memory2/1 -> Sum/3, Memory3/1
  Memory1/1 -> Sum/2, Memory2/1
  sun/1 -> Sum/1, Memory1/1

== matlab function Detumbling/Detumbling ==
  data: mag_b input double; d output double; mag_b_old input double; rate_b input double; time input double
function d = fcn(mag_b,mag_b_old,rate_b,time)
% % B-dot detumbling

if time /20 - floor(time/20) ~= 0
    x=sign(mag_b(1)-mag_b_old(1));
    y=sign(mag_b(2)-mag_b_old(2));
    z=sign(mag_b(3)-mag_b_old(3));

        if abs(rate_b(1)) > 4.5/180*pi ||abs(rate_b(2)) > 4.5/180*pi ||abs(rate_b(3)) > 4.5/180*pi 
            d=-5*[x;y;z];
        else
            d=-[x;y;z];
        end
else
    d=[0;0;0];
end

== matlab function Orbit Determination/MATLAB Function ==
  data: r1 input double; OE output double; r2 input double; r3 input double
function OE = Orbit_Determination(r1, r2, r3)
%#codegen

% Fundamental of Astrodynamics and Applications 2nd Edition
% p434 - p441のGibbs Methodを使用

MU = 3.986004418e+14;

r1xr2 = cross(r1, r2);
r2xr3 = cross(r2, r3);
r3xr1 = cross(r3, r1);

D = r1xr2 + r2xr3 + r3xr1;
N = norm(r1) * r2xr3 + norm(r2) * r3xr1 + norm(r3) * r1xr2;
S = (norm(r2) - norm(r3)) * r1 + (norm(r3) - norm(r1)) * r2 + (norm(r1) - norm(r2)) * r3;

Dxr2 = cross(D, r2);

Lg = sqrt(MU / norm(N) / norm(D));

v2 = (Dxr2 / norm(r2) + S) * Lg; 

% 以下、人工衛星の力学と制御ハンドブック p86 - p87を使用

h = cross(r2, v2);

a = 1.0 / (2.0 / norm(r2) - norm(v2)^2 / MU);
e = norm(S) / norm(D);
i = acos(h(3) / norm(h));
W = atan2(h(1), -h(2));

% eが0に近いときの場合分けを追加すること
cosE = (a - norm(r2)) / a / e;
sinE = dot(r2, v2) / e / sqrt(MU * a);
%E = atan2(sinE, cosE);
E = atan2(dot(r2, v2) * sqrt(a / MU), a - norm(r2));
M = E - e * sinE;
%costheta = (cosE - e) / (1.0 - e * cosE);
%sintheta = sqrt(1.0 - e^2) * sinE / (1.0 - e * cosE);
%theta = atan2(sintheta, costheta);
theta = atan2(sqrt(1.0 - e^2) * sinE, cosE - e);

%sinwtheta = r2(3) / norm(r2) / sin(i);
%coswtheta = (r2(1) * cos(W) + r2(2) * sin(W)) / norm(r2);
%wtheta = atan2(sinwtheta, coswtheta);
wtheta = atan2(r2(3) / sin(i), r2(1) * cos(W) + r2(2) * sin(W));
w = wtheta - theta;

OE = [a e i W w M];

== matlab function coarse kalman/MATLAB Function ==
  data: rate input double; PHI output double; dt input double
function PHI = fcn(rate,dt)
%#codegen

F = [       0 -rate(1) -rate(2) -rate(3);...
      rate(1)        0  rate(3) -rate(2);...
      rate(2) -rate(3)       0   rate(1);...
      rate(3)  rate(2) -rate(1)        0] * 0.5;

I = eye(4);

PHI = I + F * dt;

== matlab function kalman/calc_K ==
  data: Pbar input double; H input double; K output double; R input double
function K = fcn(Pbar, H, R)
%#codegen

K = (Pbar * H') / (H * Pbar * H' + R);

== matlab function kalman/calc_Pbar ==
  data: Phat input double; Pbar output double; PHI input double; Q input double
function Pbar = fcn(Phat, PHI, Q)
%#codegen

Pbar = PHI * Phat * PHI' + Q;

== matlab function kalman/calc_Phat ==
  data: K input double; H input double; Pbar input double; Phat output double
function Phat = fcn(K, H, Pbar)
%#codegen

I = eye(size(Pbar));

Phat = (I - K * H) * Pbar;

== matlab function kalman/calc_Xhat ==
  data: Xbar input double; K input double; zbar input double; H input double; Xhat output double
function Xhat = fcn(Xbar, K, zbar, H)
%#codegen

Xhat = Xbar + K * (zbar - H * Xbar);

== matlab function TRIAD/MATLAB Function ==
  data: v1 input double; v2 input double; w1 input double; w2 input double; A output double
function A = TRAID(v1, v2, w1, w2)
%#codegen

r1 = v1;
r1 = r1 / norm(r1);
r2 = cross(v1, v2);
r2 = r2 / norm(r2);
r3 = cross(r1, r2);
r3 = r3 / norm(r3);

s1 = w1;
s1 = s1 / norm(s1);
s2 = cross(w1, w2);
s2 = s2 / norm(s2);
s3 = cross(s1, s2);
s3 = s3 / norm(s3);

A = s1 * r1' + s2 * r2' + s3 * r3';

== matlab function Unloading/MomLim ==
  data: u input double; y output double; mom_lim input double
function y = mom_limit(u,mom_lim)
%#codegen

m=norm(u);

if m > mom_lim
    y=1;
else
    y=0;
end

== matlab function Unloading/RW_delta_momentum ==
  data: rate1 input double; d_H output double; rate2 input double; rate3 input double; rate4 input double; I input double; matrix_A input double
function d_H = wh_mom(rate1, rate2, rate3, rate4,I,matrix_A)
%#codegen

h1=I(1)*(rate1);h2=I(2)*(rate2);h3=I(3)*(rate3);h4=I(4)*(rate4);

d_H=matrix_A*[h1;h2;h3;h4];

== matlab function Unloading/Enable1/MATLAB Function4 ==
  data: dH input double; m output double; mag input double; max_mag input double
function m = fcn(dH,mag,max_mag)

m=1/(mag.'*mag)*cross(dH,mag);

for i=1:3
        m(i)=-sign(m(i))*max_mag;
end

% m_max=0;
% for i=1:3
%     if abs(m(i))>m_max
%         m_max=abs(m(i));
%     end
% end
% 
% m=-max_mag*m/m_max;

== matlab function sun2rate/MATLAB Function ==
  data: sun0 input double; sun1 input double; sun2 input double; rate output double; dt input double
function rate = fcn(sun0, sun1, sun2, dt)
%#codegen

if norm(sun0) * norm(sun1) * norm(sun2) == 0
    P0 = [0; 0; 0];
    P1 = [0; 0; 0];
    P2 = [0; 0; 0];
else
    P0 = sun0 / norm(sun0);
    P1 = sun1 / norm(sun1);
    P2 = sun2 / norm(sun2);
end

costheta = P0' * P1;
if costheta > 1
    costheta = 1;
end
if costheta < -1
    costheta = -1;
end
theta0 = acos(costheta);

rate0 = theta0 / dt;

if abs(rate0) < 0.1 / 180 * pi || norm(P0) * norm(P1) * norm(P2) == 0
    rate = [0; 0; 0];
else
    A = [P0'; P1'; P2'];
    d = [1; 1; 1];
    a = A\d;
    
    P01 = P1 - P0;
    P02 = P2 - P0;
    B = [P01'; P02'; a'];
    e = [0; 0; 1];
    C = B\e;
    CP0 = P0 - C;
    CP2 = P2 - C;
    CP0 = CP0 / norm(CP0);
    CP2 = CP2 / norm(CP2);
    rate = -cross(CP0, CP2) / 2.0 / dt;
end

== matlab function B2rate/MATLAB Function ==
  data: B0 input double; B1 input double; B2 input double; rate output double; dt input double
function rate = fcn(B0, B1, B2, dt)
%#codegen

if norm(B0) * norm(B1) * norm(B2) == 0
    P0 = [0; 0; 0];
    P1 = [0; 0; 0];
    P2 = [0; 0; 0];
else
    P0 = B0 / norm(B0);
    P1 = B1 / norm(B1);
    P2 = B2 / norm(B2);
end

costheta = P0' * P1;
if costheta > 1
    costheta = 1;
end
if costheta < -1
    costheta = -1;
end
theta0 = acos(costheta);

rate0 = theta0 / dt;

if abs(rate0) < 0.1 / 180 * pi || norm(P0) * norm(P1) * norm(P2) == 0
    rate = [0; 0; 0];
else
    A = [P0'; P1'; P2'];
    d = [1; 1; 1];
    a = A\d;
    
    P01 = P1 - P0;
    P02 = P2 - P0;
    B = [P01'; P02'; a'];
    e = [0; 0; 1];
    C = B\e;
    CP0 = P0 - C;
    CP2 = P2 - C;
    CP0 = CP0 / norm(CP0);
    CP2 = CP2 / norm(CP2);
    rate = -cross(CP0, CP2) / 2.0 / dt;
end

== matlab function UDdecomp ==
  data: P input double; U output double; D output double
function [U, D] = UDdecomposition(P)
%#codegen

[nProw, nPcol] = size(P);

U = zeros(nProw);
D = zeros(nProw);

for k = nProw:-1:2
    D(k,k) = P(k,k);
    U(k,k) = 1.0;
    for j = 1:k-1
        U(j,k) = P(j,k) / D(k,k);
        for i = 1:j
            P(i,j) = P(i,j) - U(i,k) * U(j,k) * D(k,k);
        end
    end
end

U(1,1) = 1.0;
D(1,1) = P(1,1);

== matlab function UDTimeUpdate ==
  data: UP input double; UP1 output double; DP1 output double; DP input double; UQ input double; DQ input double; PHI input double; x input double; x1 output double
function [UP1, DP1,x1] = UDTimeUpdate(UP,DP,UQ,DQ,PHI,x)
%#codegen

W = [PHI * UP UQ];

[nDProw,nDPcol] = size(DP);
[nDQrow,nDQcol] = size(DQ);

zero1 = zeros(nDProw, nDQcol);
zero2 = zeros(nDQrow, nDPcol);

F = [DP zero1; zero2 DQ];

[nWrow,nWcol] = size(W);

for j = nWrow:-1:2
    v = W(j,:);
    z = v * F;
    
    temp = z * v';
    DP(j,j) = temp(1,1);
    for i = 1:j
        temp = W(i,:);
        temp2 = temp * z';
        UP(i,j) = temp2(1,1) / DP(j,j);
        W(i,:) = W(i,:) - UP(i,j) * v;
    end
end

temp = W(1,:);
temp2 = temp * F * temp';
DP(1,1) = temp2(1,1);

UP1 = UP;
DP1 = DP;
x1 = PHI * x;

== matlab function CholeskyDecomposition ==
  data: R input double; sqrtR output double
function sqrtR  = CholeskyDecomp(R)
%#codegen

[nRrow, nRcol] = size(R);

sqrtR = zeros(nRrow);

for k = nRrow:-1:2
    sqrtR(k,k) = sqrt(R(k,k));
    for j = 1:k-1
        sqrtR(j,k) = R(j,k) / sqrtR(k,k);
        for i = 1:j
            R(i,j) = R(i,j) - sqrtR(i,k) * sqrtR(j,k);
        end
    end
end

sqrtR(1,1) = sqrt(R(1,1));

== matlab function Uinv ==
  data: U input double; Uinv output double
function Uinv = Uinverse(U)
%#codegen

[nUrow, nUcol] = size(U);

Uinv = zeros(nUrow);

for i = 1:nUrow
for j = 1:nUrow
    if i > j
        Uinv(i,j) = 0.0;
    elseif i == j
        Uinv(i,j) = 1.0 / U(i,j);
    else
        sum = 0.0;
        for k = i:j-1
            sum = sum + Uinv(i,k) * U(k,j);
        end
        Uinv(i,j) = -sum / U(j,j);
    end
end
end

== matlab function UDObsUpdate ==
  data: U input double; U1 output double; D1 output double; D input double; H input double; R input double; x1 output double; x input double; y input double; ObsUpdate input double
function [U1, D1, x1] = UDObsUpdate(U,D,H,R,x,y,ObsUpdate)
%#codegen

if ObsUpdate < 0.5
    U1 = U;
    D1 = D;
    x1 = x;
else
    [nUrow,nUcol] = size(U);
    
    for i = 1:nUrow
        U(i,i) = D(i,i);
    end
    
    [nHrow,nHcol] = size(H);

    FF = zeros(nHcol,1);
    GG = zeros(nHcol,1);

    for L = 1:nHrow
        y(L) = y(L) - H(L,:) * x;
        
        for j = nHcol:-1:2
            FF(j) = H(L,j) + H(L,1:j-1) * U(1:j-1,j);
            GG(j) = U(j,j) * FF(j);
        end
    
        FF(1) = H(L,1);
        GG(1) = U(1,1) * FF(1);
        alpha = R(L,L) + FF(1) * GG(1);
        gamma = 1 / alpha;
        U(1,1) = R(L,L) * gamma * U(1,1);

        for j = 2:nHcol
            beta = alpha;
            alpha = alpha + FF(j) * GG(j);
            lambda = FF(j) * gamma;
            gamma = 1 / alpha;
            U(j,j) = beta * U(j,j) * gamma;
            beta = U(1:j-1,j);

            U(1:j-1,j) = beta - lambda * GG(1:j-1);
            GG(1:j-1) = GG(1:j-1) + GG(j) * beta;
        end
        y(L) = y(L) * gamma;
        x = x + GG * y(L);
    end
    
    D1 = D;
    U1 = U;
    x1 = x;

    for i = 1:nUrow
        D1(i,i) = U1(i,i);
        U1(i,i) = 1.0;
    end
    
end

== matlab function UDUpdate ==
  data: UP input double; UP1 output double; DP1 output double; DP input double; UQ input double; DQ input double; PHI input double; x input double; x1 output double; H input double; R input double; y input double; ObsUpdate input double
function [UP1, DP1,x1] = UDUpdate(UP,DP,UQ,DQ,PHI,x,H,R,y,ObsUpdate)
%#codegen

W = [PHI * UP UQ];

[nDProw,nDPcol] = size(DP);
[nDQrow,nDQcol] = size(DQ);

zero1 = zeros(nDProw, nDQcol);
zero2 = zeros(nDQrow, nDPcol);

F = [DP zero1; zero2 DQ];

[nWrow,nWcol] = size(W);

for j = nWrow:-1:2
    v = W(j,:);
    z = v * F;
    
    temp = z * v';
    DP(j,j) = temp(1,1);
    for i = 1:j
        temp = W(i,:);
        temp2 = temp * z';
        UP(i,j) = temp2(1,1) / DP(j,j);
        W(i,:) = W(i,:) - UP(i,j) * v;
    end
end

temp = W(1,:);
temp2 = temp * F * temp';
DP(1,1) = temp2(1,1);

UP1 = UP;
DP1 = DP;
x1 = PHI * x;

if ObsUpdate > 0.5

    U = UP1;
    D = DP1;
    x = x1;
    
    [nUrow,nUcol] = size(U);
    
    for i = 1:nUrow
        U(i,i) = D(i,i);
    end

    [nHrow,nHcol] = size(H);

    FF = zeros(nHcol,1);
    GG = zeros(nHcol,1);

    for L = 1:nHrow
        y(L) = y(L) - H(L,:) * x;
        
        for j = nHcol:-1:2
            FF(j) = H(L,j) + H(L,1:j-1) * U(1:j-1,j);
            GG(j) = U(j,j) * FF(j);
        end
        
        FF(1) = H(L,1);
        GG(1) = U(1,1) * FF(1);
        alpha = R(L,L) + FF(1) * GG(1);
        gamma = 1 / alpha;
        U(1,1) = R(L,L) * gamma * U(1,1);

        for j = 2:nHcol
            beta = alpha;
            alpha = alpha + FF(j) * GG(j);
            lambda = FF(j) * gamma;
            gamma = 1 / alpha;
            U(j,j) = beta * U(j,j) * gamma;
            beta = U(1:j-1,j);

            U(1:j-1,j) = beta - lambda * GG(1:j-1);
            GG(1:j-1) = GG(1:j-1) + GG(j) * beta;
        end
        y(L) = y(L) * gamma;
        x = x + GG * y(L);
    end

    DP1 = D;
    UP1 = U;
    x1 = x;
    
    for i = 1:nUrow
        DP1(i,i) = U(i,i);
        UP1(i,i) = 1.0;
    end
    
end

== matlab function Unloading/RateLim ==
  data: u input double; y output double; Rate_lim input double
function y = Rate_limit(u,Rate_lim)
%#codegen

m=abs(u(1));

if m < abs(u(2))
    m=abs(u(2));
end
if m < abs(u(3))
    m=abs(u(3));
end
if m < abs(u(4))
    m=abs(u(4));
end

if m > Rate_lim
    y=1;
else
    y=0;
end

== matlab function Unloading/body_delta_momentum ==
  data: rate input double; d_H output double; I input double; rate_t input double
function d_H = body_mom(rate,I,rate_t)
%#codegen

d_H=I*(rate_t-rate);

== matlab function trigger_box ==
  data: clock input double; m_t output double; c_t output double; m_d input double; rest input double; cont_d input double
function [m_t,c_t] = trigger(clock,m_d,rest,cont_d)
%#codegen

% m_d=5;%measure_duration
% rest=1;%MTQ_effect
% cont_d=4*60;%cont_duration
cont_p=m_d+rest+cont_d;%cont_period

    m_t=0;
    c_t=0;

if clock-floor(clock/cont_p)*cont_p <= m_d && clock-floor(clock/cont_p)*cont_p >= rest 
    m_t = 1; % measurement trig
elseif clock-floor(clock/cont_p)*cont_p > m_d
    c_t = 1; % control trig
end

== matlab function coarse kalman/MATLAB Function1 ==
  data: q input double; H output double; m input double; s input double
function H = fcn(q,m,s)
%#codegen

q0 = q(1);
q1 = q(2);
q2 = q(3);
q3 = q(4);
mx = m(1);
my = m(2);
mz = m(3);
sx = s(1);
sy = s(2);
sz = s(3);

% H = [(2*q0*mx + q3*my - q2*mz) (2*q1*mx + q2*my + q3*mz) (q1*my - q0*mz) (q0*my + q1*mz); ...
%          (-q3*mx + 2*q0*my + q1*mz) (q2*mx + q0*mz) (q1*mx + 2*q2*my + q3*mz) (-q0*mx + q2*mz); ...
%          (q2*mx - q1*my + 2*q0*mz) (q3*mx - q0*my) (q0*mx - q3*my) (q1*mx + q2*my + 2*q3*mz); ...
%          (2*q0*sx + q3*sy - q2*sz) (2*q1*sx + q2*sy + q3*sz) (q1*sy - q0*sz) (q0*sy + q1*sz); ...
%          (-q3*sx + 2*q0*sy + q1*sz) (q2*sx + q0*sz) (q1*sx + 2*q2*sy + q3*sz) (-q0*sx + q2*sz); ...
%          (q2*sx - q1*sy + 2*q0*sz) (q3*sx - q0*sy) (q0*sx - q3*sy) (q1*sx + q2*sy + 2*q3*sz)];

H = [( q0*mx+q3*my-q2*mz) (q1*mx+q2*my+q3*mz) (-q2*mx+q1*my-q0*mz) (-q3*mx+q0*my+q1*mz); ...
     (-q3*mx+q0*my+q1*mz) (q2*mx-q1*my+q0*mz) ( q1*mx+q2*my+q3*mz) (-q0*mx-q3*my+q2*mz); ...
     ( q2*mx-q1*my+q0*mz) (q3*mx-q0*my-q1*mz) ( q0*mx+q3*my-q2*mz) ( q1*mx+q2*my+q3*mz); ...
     ( q0*sx+q3*sy-q2*sz) (q1*sx+q2*sy+q3*sz) (-q2*sx+q1*sy-q0*sz) (-q3*sx+q0*sy+q1*sz); ...
     (-q3*sx+q0*sy+q1*sz) (q2*sx-q1*sy+q0*sz) ( q1*sx+q2*sy+q3*sz) (-q0*sx-q3*sy+q2*sz); ...
     ( q2*sx-q1*sy+q0*sz) (q3*sx-q0*sy-q1*sz) ( q0*sx+q3*sy-q2*sz) ( q1*sx+q2*sy+q3*sz)] * 2.0;

== matlab function coarse kalman/MATLAB Function2 ==
  data: y output double; s input double
function y = fcn(s)
%#codegen

y = 1;

if s(1) > 2
    y = 0;
end

== matlab function calc sun pointing/MATLAB Function1 ==
  data: R input double; n1 output double; V input double; S input double; n2 output double; y output double; z output double
function [n1,n2,y,z] = fcn(R, V, S)
%#codegen

n1 = -cross(R,V);
n1 = n1 / norm(n1);

nsun = S / norm(S);
n2 = -(nsun - (nsun' * n1) * n1);
n2 = n2 / norm(n2);

y = [0; 1; 0];
z = [0; 0; 1];

== matlab function orbit determination/MATLAB Function ==
  data: u input double; y output double
function y = fcn(u)
%#codegen

y = 0;

if u(1) || u(2) || u(3)
    y = 1;
end

== matlab function orbit determination/UDUpdate ==
  data: UP input double; UP1 output double; DP1 output double; DP input double; UQ input double; DQ input double; PHI input double; x input double; x1 output double; H input double; R input double; y input double; ObsUpdate input double
function [UP1, DP1,x1] = UDUpdate(UP,DP,UQ,DQ,PHI,x,H,R,y,ObsUpdate)
%#codegen

W = [PHI * UP UQ];

[nDProw,nDPcol] = size(DP);
[nDQrow,nDQcol] = size(DQ);

zero1 = zeros(nDProw, nDQcol);
zero2 = zeros(nDQrow, nDPcol);

F = [DP zero1; zero2 DQ];

[nWrow,nWcol] = size(W);

for j = nWrow:-1:2
    v = W(j,:);
    z = v * F;
    
    temp = z * v';
    DP(j,j) = temp(1,1);
    for i = 1:j
        temp = W(i,:);
        temp2 = temp * z';
        UP(i,j) = temp2(1,1) / DP(j,j);
        W(i,:) = W(i,:) - UP(i,j) * v;
    end
end

temp = W(1,:);
temp2 = temp * F * temp';
DP(1,1) = temp2(1,1);

UP1 = UP;
DP1 = DP;
x1 = PHI * x;

if ObsUpdate > 0.5

    U = UP1;
    D = DP1;
    x = x1;
    
    [nUrow,nUcol] = size(U);
    
    for i = 1:nUrow
        U(i,i) = D(i,i);
    end

    [nHrow,nHcol] = size(H);

    FF = zeros(nHcol,1);
    GG = zeros(nHcol,1);

    for L = 1:nHrow
        y(L) = y(L) - H(L,:) * x;
        
        for j = nHcol:-1:2
            FF(j) = H(L,j) + H(L,1:j-1) * U(1:j-1,j);
            GG(j) = U(j,j) * FF(j);
        end
        
        FF(1) = H(L,1);
        GG(1) = U(1,1) * FF(1);
        alpha = R(L,L) + FF(1) * GG(1);
        gamma = 1 / alpha;
        U(1,1) = R(L,L) * gamma * U(1,1);

        for j = 2:nHcol
            beta = alpha;
            alpha = alpha + FF(j) * GG(j);
            lambda = FF(j) * gamma;
            gamma = 1 / alpha;
            U(j,j) = beta * U(j,j) * gamma;
            beta = U(1:j-1,j);

            U(1:j-1,j) = beta - lambda * GG(1:j-1);
            GG(1:j-1) = GG(1:j-1) + GG(j) * beta;
        end
        y(L) = y(L) * gamma;
        x = x + GG * y(L);
    end

    DP1 = D;
    UP1 = U;
    x1 = x;
    
    for i = 1:nUrow
        DP1(i,i) = U(i,i);
        UP1(i,i) = 1.0;
    end
    
end

== matlab function orbit determination/UDdecomp1 ==
  data: P input double; U output double; D output double
function [U, D] = UDdecomposition(P)
%#codegen

[nProw, nPcol] = size(P);

U = zeros(nProw);
D = zeros(nProw);

for k = nProw:-1:2
    D(k,k) = P(k,k);
    U(k,k) = 1.0;
    for j = 1:k-1
        U(j,k) = P(j,k) / D(k,k);
        for i = 1:j
            P(i,j) = P(i,j) - U(i,k) * U(j,k) * D(k,k);
        end
    end
end

U(1,1) = 1.0;
D(1,1) = P(1,1);

== matlab function orbit determination/calc PHI ==
  data: rIJK input double; PHI output double; dt input double
function PHI = fcn(rIJK, dt)
%#codegen

GE = 3.986004415e+5; % km^3/s^2

x = rIJK(1);
y = rIJK(2);
z = rIJK(3);
r = sqrt(x^2 + y^2 + z^2);

% % if r < 1.0e-6
% %     F = [0 0 0 0 0 0; ...
% %          0 0 0 0 0 0; ...
% %          0 0 0 0 0 0; ...
% %          0 0 0 0 0 0; ...
% %          0 0 0 0 0 0; ...
% %          0 0 0 0 0 0];
% % else
% % 
% %     F11 = GE / r^3 * (-1.0 + 3.0 * GE * x^2 / r^2);
% %     F22 = GE / r^3 * (-1.0 + 3.0 * GE * y^2 / r^2);
% %     F33 = GE / r^3 * (-1.0 + 3.0 * GE * z^2 / r^2);
% %     F12 = 3.0 * GE * x * y / r^5;
% %     F13 = 3.0 * GE * x * z / r^5;
% %     F23 = 3.0 * GE * y * z / r^5;
% % 
% %     F = [0 0 0 1 0 0; ...
% %          0 0 0 0 1 0; ...
% %          0 0 0 0 0 1; ...
% %          F11 F12 F13 0 0 0; ...
% %          F12 F22 F23 0 0 0; ...
% %          F13 F23 F33 0 0 0];
% % 
% % end
% % 
% % I = eye(size(F));
% % 
% % PHI = I + F * dt + F^2 / 2.0 * dt^2 + F^3 / 6.0 * dt^3 + F^4 / 24.0 * dt^4;
% 
% PHI11 = 1.0 + GE * dt^2 / 2.0 / r^3 * (3.0 * x^2 / r^2 - 1.0);
% PHI12 = 3.0 * GE * dt^2 * x * y / 2.0 / r^5;
% PHI13 = 3.0 * GE * dt^2 * x * z / 2.0 / r^5;
% PHI21 = PHI12;
% PHI22 = 1.0 + GE * dt^2 / 2.0 / r^3 * (3.0 * y^2 / r^2 - 1.0);
% PHI23 = 3.0 * GE * dt^2 * y * z / 2.0 / r^5;
% PHI31 = PHI13;
% PHI32 = PHI23;
% PHI33 = 1.0 + GE * dt^2 / 2.0 / r^3 * (3.0 * z^2 / r^2 - 1.0);
% PHI41 = GE * dt / r^3 * (3.0 * x^2 / r^2 - 1.0);
% PHI42 = 3.0 * GE * dt * x * y / r^5;
% PHI43 = 3.0 * GE * dt * x * z / r^5;
% PHI51 = PHI42;
% PHI52 = GE * dt / r^3 * (3.0 * y^2 / r^2 - 1.0);
% PHI53 = 3.0 * GE * dt * y * z / r^5;
% PHI61 = PHI43;
% PHI62 = PHI53;
% PHI63 = GE * dt / r^3 * (3.0 * z^2 / r^2 - 1.0);
% 
% PHI = [PHI11 PHI12 PHI13 dt 0 0; ...
%        PHI21 PHI22 PHI23 0 dt 0; ...
%        PHI31 PHI32 PHI33 0 0 dt; ...
%        PHI41 PHI42 PHI43 1 0 0; ...
%        PHI51 PHI52 PHI53 0 1 0; ...
%        PHI61 PHI62 PHI63 0 0 1];
% 
% I = eye(size(PHI));

G = [0 0 0 1 0 0;
     0 0 0 0 1 0;
     0 0 0 0 0 1;
     -GE / r^3 0 0 0 0 0;
     0 -GE / r^3 0 0 0 0;
     0 0 -GE / r^3 0 0 0];
 
F11 = GE / r^3 * (-1.0 + 3.0 * x^2 / r^2);
F22 = GE / r^3 * (-1.0 + 3.0 * y^2 / r^2);
F33 = GE / r^3 * (-1.0 + 3.0 * z^2 / r^2);
F12 = 3.0 * GE * x * y / r^5;
F13 = 3.0 * GE * x * z / r^5;
F23 = 3.0 * GE * y * z / r^5;

F = [0 0 0 1 0 0; ...
     0 0 0 0 1 0; ...
     0 0 0 0 0 1; ...
     F11 F12 F13 0 0 0; ...
     F12 F22 F23 0 0 0; ...
     F13 F23 F33 0 0 0];
I = eye(size(F));

PHI = I + F * dt + F^2 * dt^2 / 2 + F^3 * dt^3 / 6.0 + F^4 * dt^4 / 24.0;
PHI = I + G * dt + G^2 * dt^2 / 2 + G^3 * dt^3 / 6.0 + G^4 * dt^4 / 24.0;
   
if r < 1e-6
    PHI = I;
end

== matlab function attitude determination/MATLAB Function ==
  data: u input double; y output double; e input double
function y = fcn(u,e)
%#codegen

y = 0;

if u(1) || u(2) || u(3) || u(4)
    y = 1;
end

if e
    y = 0;
end

== matlab function attitude determination/CholeskyDecomposition ==
  data: R input double; sqrtR output double
function sqrtR  = CholeskyDecomp(R)
%#codegen

[nRrow, nRcol] = size(R);

sqrtR = zeros(nRrow);

for k = nRrow:-1:2
    sqrtR(k,k) = sqrt(R(k,k));
    for j = 1:k-1
        sqrtR(j,k) = R(j,k) / sqrtR(k,k);
        for i = 1:j
            R(i,j) = R(i,j) - sqrtR(i,k) * sqrtR(j,k);
        end
    end
end

sqrtR(1,1) = sqrt(R(1,1));
